simulink model "mod_v1"  (R2022b)
settings: Solver=VariableStepAuto  StartTime=0.0  StopTime=250  RelTol=1e-3
values from neighbouring files (symbols this model uses):
  attrito = Thrust*0.01    [data.m]
  C_D = 0.029    [data.m]    (also in data_tom(OLD).m = 0.024)
  C_L = 0.5639    [data.m]
  massa = 20    [data.m]
  peso = massa*9.8    (= 196)    [data.m]
  Thrust = D    (= 10.080254275)    [data.m]    (also in data_tom(OLD).m = D)
undefined symbols (not defined in the file or in its folder): magnitude
settings Model: Creator=tomde  LastModifiedBy=tomde

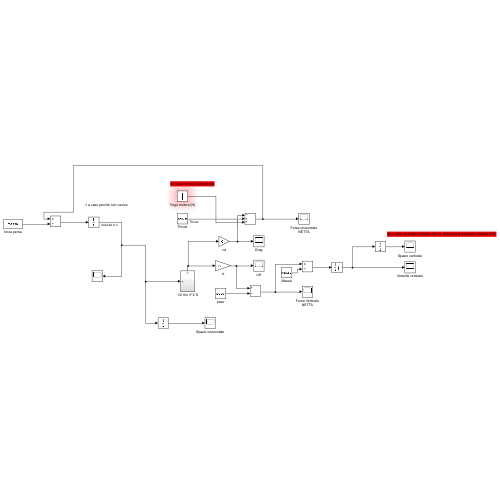
[thumbnail: Simulink's stored preview of the top-level diagram]
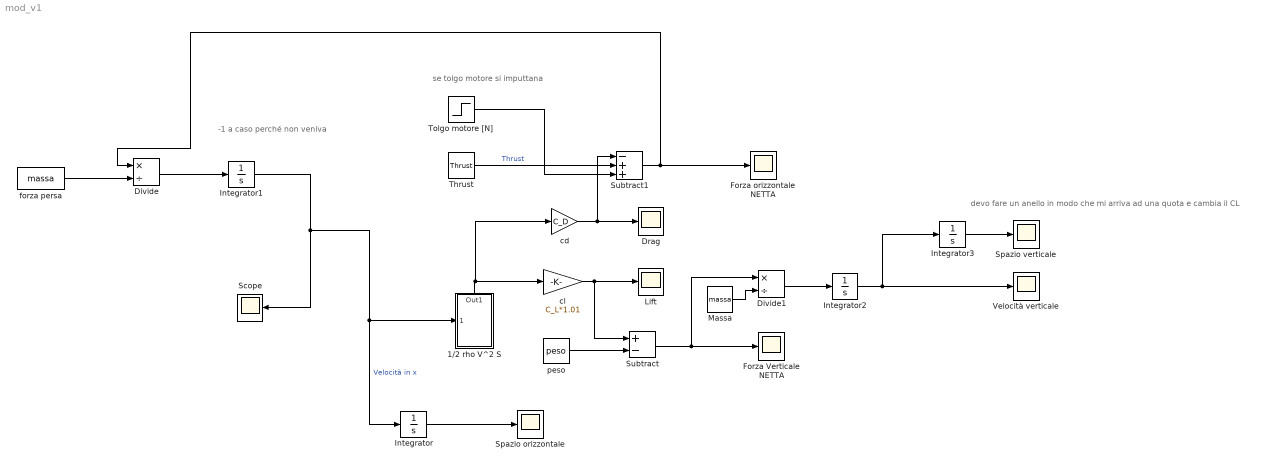
== system mod_v1 ==
  note: -1 a caso perché non veniva
  note: devo fare un anello in modo che mi arriva ad una quota e cambia il CL
  note: se tolgo motore si imputtana
  1/2 rho V^2 S : Subsystem
      settings: PortSchema="{\"entries\":[{\"content\":{\"sides\":[{\"content\":{\"connectorIds\":[\"In1\"]},\"type\":\"ConnectorPlacement.EquallySpacedRectSide\",\"uuid\":\"8dba6aa6-7766-45aa-86ae-97b1773e1631\"},{\"content\":{\"connectorIds\":[],\"side\":\"RIGHT\"},\"type\":\"ConnectorPlacement.EquallySpacedRectSide\",\"uuid\":\"4ac2620c-8d2a-4351-9341-7ca9103b5b04\"},{\"content\":{\"connectorIds\":[\"Out1\"],\"side\":\"TOP\"},\"type\":\"ConnectorPlacement.EquallySpacedRectSide\",\"uuid\":\"f1b59344-80b4-4e38-ac91-c424da8eb23a\"}]},\"type\":\"ConnectorPlacement.EquallySpacedConnector\",\"uuid\":\"f854a4ba-39db-402c-825c-471c05348acc\"}],\"packageUris\":[\"http://schema.mathworks.com/mf0/Connector/R2020b\"],\"version\":\"1.0\"}"
  Divide : Product  Inputs=*/
  Divide1 : Product  Inputs=*/
  Drag : Scope
  Forza Verticale NETTA : Scope
  Forza orizzontale NETTA : Scope
  Integrator : Integrator
  Integrator1 : Integrator
  Integrator2 : Integrator  LimitOutput=on  LowerSaturationLimit=0
  Integrator3 : Integrator
  Lift : Scope
  Massa : Constant  Value=massa
  Scope : Scope
  Spazio orizzontale : Scope
  Spazio verticale : Scope
  Subtract : Sum  Inputs=+-
  Subtract1 : Sum  Inputs=-++
  Thrust : Constant  Value=Thrust
  Tolgo motore [N] : Step  Time=attrito  After=-Thrust  SampleTime=0
  Velocità verticale : Scope
  cd : Gain  Gain=C_D
  cl : Gain  Gain=C_L*1.01
  forza persa : Constant  Value=massa
  peso : Constant  Value=peso
  wires:
  1/2 rho V^2 S/1(Out1) -> cd/1, cl/1
  cl/1 -> Subtract/1, Lift/1
  cd/1 -> Subtract1/1, Drag/1
  Integrator/1 -> Spazio orizzontale/1
  peso/1 -> Subtract/2
  Subtract/1 -> Divide1/1, Forza Verticale NETTA/1
  Subtract1/1 -> Divide/1, Forza orizzontale NETTA/1
  forza persa/1 -> Divide/2
  Massa/1 -> Divide1/2
  Divide1/1 -> Integrator2/1
  Integrator2/1 -> Integrator3/1, Velocità verticale/1
  Divide/1 -> Integrator1/1
  Integrator1/1 -> Scope/1, Integrator/1, 1/2 rho V^2 S/1(In1)  "Velocità in x"
  Thrust/1 -> Subtract1/2  "Thrust"
  Integrator3/1 -> Spazio verticale/1
  Tolgo motore [N]/1 -> Subtract1/3

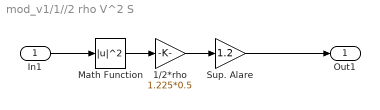
== system mod_v1/1//2 rho V^2 S ==
  In1 : Inport
  1/2*rho : Gain  Gain=1.225*0.5
  Math Function : Math  Operator=magnitude^2  OutputSignalType=real
  Sup. Alare : Gain  Gain=1.2
  Out1 : Outport
  wires:
  Math Function/1 -> 1/2*rho/1
  In1/1 -> Math Function/1
  Sup. Alare/1 -> Out1/1
  1/2*rho/1 -> Sup. Alare/1
